simulink model "model_Electrolyzer_battery_Generator"  (R2021b)
settings: Solver=VariableStepAuto  StartTime=0.0  StopTime=30  RelTol=1e-3
values from neighbouring files (symbols this model uses):
  D5 = 1.5/100/(0.01*F0)*1    (= 0.03)    [runSimulations_Nordic_GB_HVDC.m]
  F0 = 50    [runSimulations_Nordic_GB_HVDC.m]
  H_0 = 214750.0    (= 214750)    [runSimulations_Nordic_GB_HVDC.m]
  P_D5 = 37500*0    (= 0)    [runSimulations_Nordic_GB_HVDC.m]
  Ploss = 1792.5    [runSimulations_Nordic_GB_HVDC.m]
  re = 399.9998999999987    (= 399.9999)    [runSimulations_Nordic_GB_HVDC.m]
  rg = 478.33333333333337    (= 478.333333333)    [runSimulations_Nordic_GB_HVDC.m]
  rh = 914.166766666668    (= 914.166766667)    [runSimulations_Nordic_GB_HVDC.m]
  rs = 0.0    (= 0)    [runSimulations_Nordic_GB_HVDC.m]
  te = 0.2    [runSimulations_Nordic_GB_HVDC.m]
  tg = 15    [runSimulations_Nordic_GB_HVDC.m]
  th = 0.2    [runSimulations_Nordic_GB_HVDC.m]
  ts = 0.2    [runSimulations_Nordic_GB_HVDC.m]
libraries: simulink x4
settings Model: Creator=jcastano  LastModifiedBy=jcastano

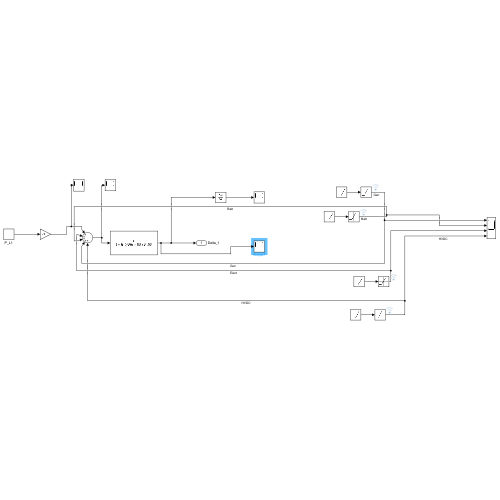
[thumbnail: Simulink's stored preview of the top-level diagram]
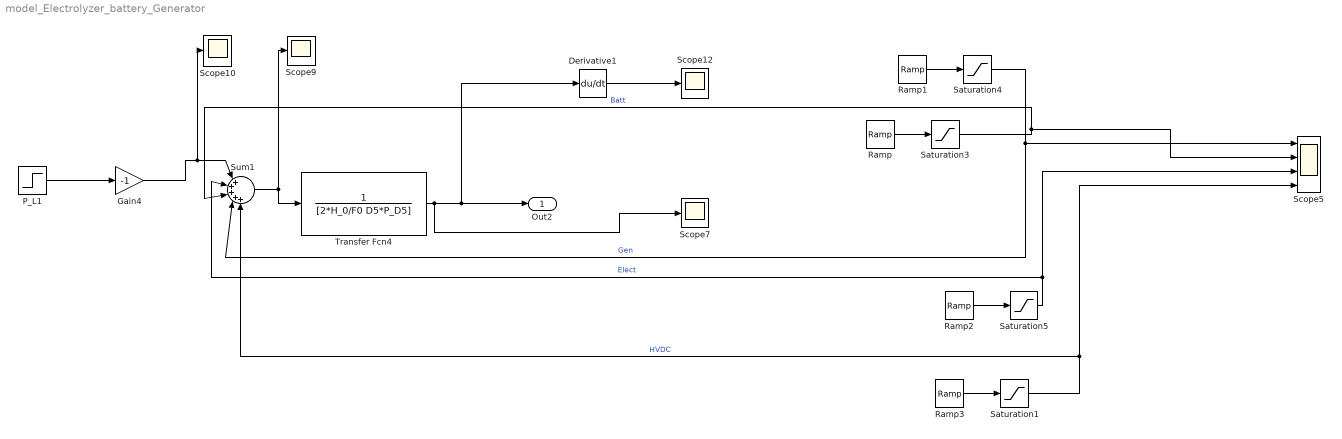
== system model_Electrolyzer_battery_Generator ==
  Derivative1 : Derivative
  Gain4 : Gain  Gain=-1
  P_L1 : Step  Time=0  Before=Ploss  After=Ploss  SampleTime=0
  Ramp : simulink/Sources/Ramp  slope=rs/ts  start=0  InitialOutput=0
  Ramp1 : simulink/Sources/Ramp  slope=rg/tg  start=0  InitialOutput=0
  Ramp2 : simulink/Sources/Ramp  slope=re/te  start=0  InitialOutput=0
  Ramp3 : simulink/Sources/Ramp  slope=rh/th  start=0  InitialOutput=0
  Saturation1 : Saturate  UpperLimit=rh  LowerLimit=0
  Saturation3 : Saturate  UpperLimit=rs  LowerLimit=0
  Saturation4 : Saturate  UpperLimit=rg  LowerLimit=0
  Saturation5 : Saturate  UpperLimit=re  LowerLimit=0
  Scope{7,9..10,12} (4 alike) : Scope
  Scope5 : Scope  NumInputPorts=4
  Sum1 : Sum  Inputs=|+++++
  Transfer Fcn4 : TransferFcn  Denominator=[2*H_0/F0 D5*P_D5]
  Out2 : Outport  SignalName=Delta_f
  wires:
  Ramp/1 -> Saturation3/1
  Ramp1/1 -> Saturation4/1
  Ramp2/1 -> Saturation5/1
  P_L1/1 -> Gain4/1
  Saturation3/1 -> Scope5/2, Sum1/3  "Batt"
  Saturation4/1 -> Scope5/1, Sum1/4  "Gen"
  Sum1/1 -> Scope9/1, Transfer Fcn4/1
  Transfer Fcn4/1 -> Scope7/1, Derivative1/1, Out2/1
  Gain4/1 -> Scope10/1, Sum1/1
  Saturation5/1 -> Scope5/3, Sum1/2  "Elect"
  Derivative1/1 -> Scope12/1
  Ramp3/1 -> Saturation1/1
  Saturation1/1 -> Scope5/4, Sum1/5  "HVDC"
